simulink model "Final_Report_Carrieri"  (R2020b)
settings: Solver=VariableStepAuto  StartTime=0.0  StopTime=10.0  MaxStep=0.5e-4  RelTol=1e-3
libraries: nesl_utility x12, fl_lib x10, ee_lib x9, simulink x2, powerlib x1
settings Model: Creator=claudio.rossi  LastModifiedBy=lapoc
settings SolverCC: ZeroCrossAlgorithm=Adaptive
settings DebuggingCC: IgnoredZcDiagnostic=none
settings SFSimCC: CustomCodeUndefinedFunction=UseInterfaceOnly

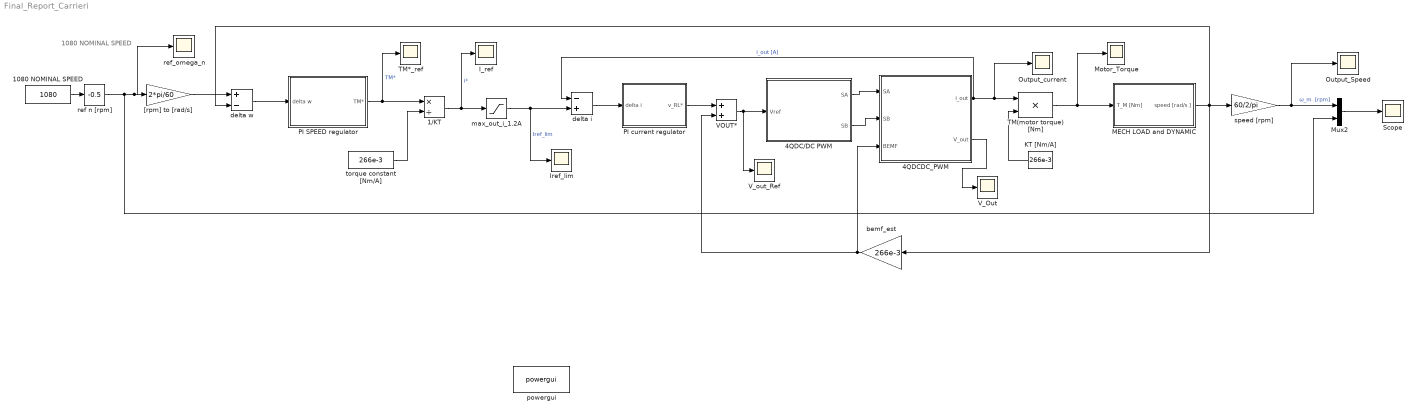
== system Final_Report_Carrieri ==
  note: 1080 NOMINAL SPEED
  1/KT : Product  Inputs=*/
  1080 NOMINAL SPEED : Constant  Value=1080
  4QDC/DC PWM : Subsystem
  4QDCDC_PWM : Subsystem
  I_ref : Scope
  Iref_lim : Scope
  KT [Nm/A] : Constant  Value=266e-3
  MECH LOAD and DYNAMIC : Subsystem
  Motor_Torque : Scope
  Mux2 : Mux  Inputs=2
  Output_Speed : Scope
  Output_current : Scope
  PI SPEED regulator : Subsystem
  PI current regulator : Subsystem
  Scope : Scope
  TM(motor torque) [Nm] : Product
  TM*_ref : Scope
  VOUT* : Sum
  V_Out : Scope
  V_out_Ref : Scope
  "[rpm] to [rad/s]" : Gain  Gain=2*pi/60
  bemf_est : Gain  Gain=266e-3
  delta i : Sum  Inputs=-+
  delta w : Sum  Inputs=+-
  max_out_i_1.2A : Saturate  UpperLimit=1.2  LowerLimit=-1.2
  powergui : powerlib/powergui  Priority=1  SimulationMode=Continuous  SampleTime=50e-6  frequency=60  Iterations=50  frequencyindice=60  Pbase=100e6  ErrMax=1e-4  UnitsV=kV  UnitsW=MW  buscounter=0  FunctionMessages=off  echomessages=off  EnableUseOfTLC=off  CurrentSourceSwitches=off  DisableSnubberDevices=off  DisableRonSwitches=off  DisableVfSwitches=off  DisplayEquations=off  AutomaticDiscreteSolvers=off  SolverType=Tustin/Backward Euler (TBE)  Interpol=off  ExternalGateDelay=off  methode=off  Ts=100  x0status=blocks  SPID=on  SwTol=0  HookPort=off  NonlinearTolerance=1e-4  nMaxIteration=100  ContinueOnMaxIteration=off  RestoreLinks=warning  ResistiveCurrentMeasurement=off  Frange=[0:2:500]  Ylog=off  Xlog=on  ShowGrid=off  save=off  variable=ZData  structure=0  ZoomFFT=off  StartTime=0.0  cycles=1  DisplayStyle=1  fundamental=60  FreqAxis=off  MaxFrequency=1000  frequencyindicesteady=1  RmsSteady=1  display=off
  ref n [rpm] : simulink/Math Operations/Slider Gain  gain=-0.5  low=-1  high=1
  ref_omega_n : Scope
  speed [rpm] : Gain  Gain=60/2/pi
  torque constant [Nm/A] : Constant  Value=266e-3
  wires:
  TM(motor torque) [Nm]/1 -> Motor_Torque/1, MECH LOAD and DYNAMIC/1(T_M [Nm])
  max_out_i_1.2A/1 -> Iref_lim/1, delta i/2  "Iref_lim"
  VOUT*/1 -> V_out_Ref/1, 4QDC/DC PWM/1(Vref)
  ref n [rpm]/1 -> "[rpm] to [rad/s]"/1, ref_omega_n/1, Mux2/2
  Mux2/1 -> Scope/1
  4QDC/DC PWM/2(SB) -> 4QDCDC_PWM/2(SB)
  4QDC/DC PWM/1(SA) -> 4QDCDC_PWM/1(SA)
  KT [Nm/A]/1 -> TM(motor torque) [Nm]/2
  1080 NOMINAL SPEED/1 -> ref n [rpm]/1
  4QDCDC_PWM/2(V_out) -> V_Out/1
  4QDCDC_PWM/1(i_out) -> delta i/1, Output_current/1, TM(motor torque) [Nm]/1  "i_out [A]"
  speed [rpm]/1 -> Output_Speed/1, Mux2/1  "ω_m  [rpm]"
  1/KT/1 -> max_out_i_1.2A/1, I_ref/1  "i*"
  torque constant [Nm/A]/1 -> 1/KT/2
  "[rpm] to [rad/s]"/1 -> delta w/1
  PI SPEED regulator/1(TM*) -> TM*_ref/1, 1/KT/1  "TM*"
  MECH LOAD and DYNAMIC/1(speed [rad/s ]) -> bemf_est/1, speed [rpm]/1, delta w/2
  delta w/1 -> PI SPEED regulator/1(delta w)
  bemf_est/1 -> VOUT*/2, 4QDCDC_PWM/3(BEMF)
  delta i/1 -> PI current regulator/1(delta i)
  PI current regulator/1(v_RL*) -> VOUT*/1

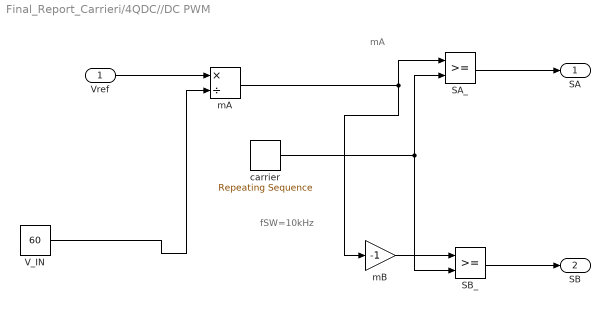
== system Final_Report_Carrieri/4QDC//DC PWM ==
  note: fSW=10kHz
  note: mA
  Vref : Inport
  SA_ : RelationalOperator  OutDataTypeStr=boolean  RndMeth=Simplest
  SB_ : RelationalOperator  OutDataTypeStr=boolean  RndMeth=Simplest
  V_IN : Constant  Value=60
  carrier : simulink/Sources/Repeating Sequence  rep_seq_t=[0 1e-4/2 1e-4]  rep_seq_y=[-1 1 -1]
  mA : Product  Inputs=*/
  mB : Gain  Gain=-1
  SA : Outport  VectorParamsAs1DForOutWhenUnconnected=off
  SB : Outport  Port=2  VectorParamsAs1DForOutWhenUnconnected=off
  wires:
  V_IN/1 -> mA/2
  Vref/1 -> mA/1
  carrier/1 -> SB_/2, SA_/2
  SB_/1 -> SB/1
  mA/1 -> mB/1, SA_/1
  mB/1 -> SB_/1
  SA_/1 -> SA/1

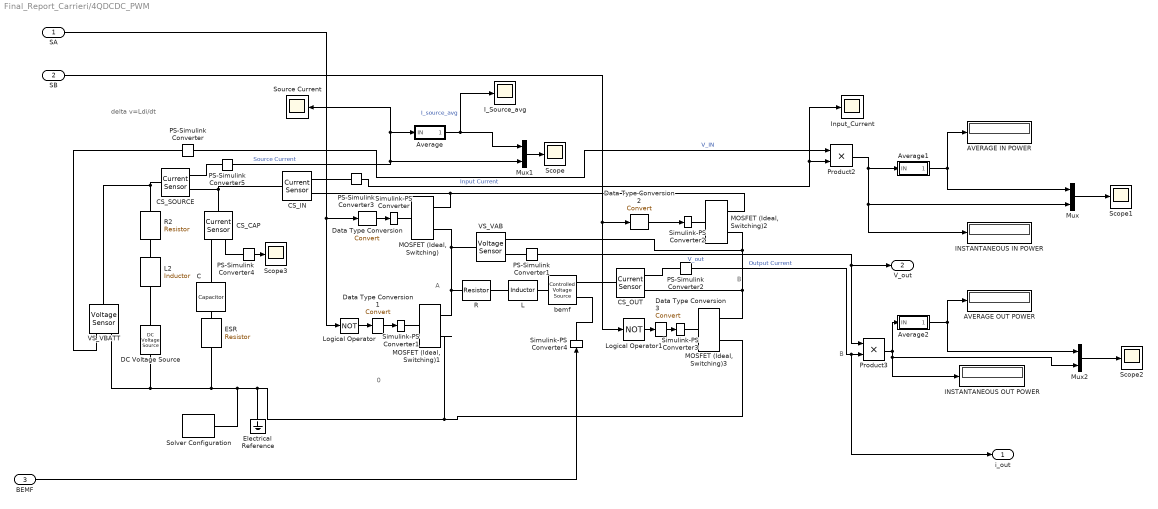
== system Final_Report_Carrieri/4QDCDC_PWM ==
  note: delta v=Ldi/dt
  note: B
  note: 0
  note: A
  note: B
  SA : Inport
  SB : Inport  Port=2
  BEMF : Inport  Port=3
  AVERAGE IN POWER : Display
  AVERAGE OUT POWER : Display
  Average : Subsystem  mask{Ts=1e-4/2}
      mask prompts: Ts "period"
  Average1 : Subsystem  mask{Ts=1e-4/2}
      mask prompts: Ts "period"
  Average2 : Subsystem  mask{Ts=1e-4/2}
      mask prompts: Ts "period"
  C : fl_lib/Electrical/Electrical Elements/Capacitor  c=10 mF  r=1e-9 Ohm  g=0 1/Ohm  i_specify=off  i_priority=None  i=0 A  i_nominal_specify=off  i_nominal_unit=A  i_nominal_value=1  v_specify=off  v_priority=None  v=0 V  v_nominal_specify=off  v_nominal_unit=V  v_nominal_value=1  vc_specify=off  vc_priority=High  vc=0 V  vc_nominal_specify=off  vc_nominal_unit=V  vc_nominal_value=1
  CS_CAP : fl_lib/Electrical/Electrical Sensors/Current Sensor
  CS_IN : fl_lib/Electrical/Electrical Sensors/Current Sensor
  CS_OUT : fl_lib/Electrical/Electrical Sensors/Current Sensor
  CS_SOURCE : fl_lib/Electrical/Electrical Sensors/Current Sensor
  DC Voltage Source : fl_lib/Electrical/Electrical Sources/DC Voltage Source  v0=60 V
  Data Type Conversion{,1..3} (4 alike) : DataTypeConversion
  ESR : ee_lib/Passive/Resistor  R=0.01 Ohm  R_tol=5  enable_R_tol=0  tol_distribution=1  nSigma=4  enable_operating_limits=0  operating_limit_action=2  max_working_voltage=100 V  power_rating=1 W  enable_faults=0  fault_action=1  R_faulted=inf Ohm  enable_temporal_fault=0  t_fault=1 s  enable_behavioral_fault=0  max_permissible_current=1 A  t_fail_on_current=1 s  noise_mode=0  sample_time=1e-3 s  repeatability=1  auto_seed=3499211588  user_seed=0  Tdevice=25 degC  alpha=3.93e-3 1/K  Tmeas=25 degC  thermal_mass=100 J/K  power_derating_T1=70 degC  power_derating_T2=155 degC  operating_temperature_range_vec=[-50, 150] degC  temperature_specify=off  temperature_priority=High  temperature=298.15 K  temperature_nominal_specify=off  temperature_nominal_unit=K  temperature_nominal_value=1
  Electrical Reference : fl_lib/Electrical/Electrical Elements/Electrical Reference
  INSTANTANEOUS IN POWER : Display
  INSTANTANEOUS OUT POWER : Display
  I_Source_avg : Scope
  Input_Current : Scope
  L : ee_lib/Passive/Inductor  l=6.4e-3 H  L_tol=20  enable_L_tol=0  tol_distribution=1  nSigma=4  r=0 Ohm  g=1e-9 1/Ohm  enable_operating_limits=0  operating_limit_action=2  max_working_current=1 A  power_rating=1 W  enable_faults=0  fault_action=1  lambdaPercent=50  k_faulted=0.9999  turnsShort=0  openCct=0  groundShort=0  groundShortG=0 1/Ohm  tau_fault=1e-3 s  enable_temporal_fault=0  t_fault=1 s  enable_behavioral_fault=0  max_permissible_voltage=100 V  n_fail_on_voltage=1  max_permissible_current=1 A  t_fail_on_current=1 s  i_L_specify=off  i_L_priority=High  i_L=0 A  i_L_nominal_specify=off  i_L_nominal_unit=A  i_L_nominal_value=1
  L2 : ee_lib/Passive/Inductor  l=0.6 mH  L_tol=5  enable_L_tol=0  tol_distribution=1  nSigma=4  r=0 Ohm  g=1e-6 1/Ohm  enable_operating_limits=0  operating_limit_action=2  max_working_current=1 A  power_rating=1 W  enable_faults=0  fault_action=1  lambdaPercent=50  k_faulted=0.9999  turnsShort=0  openCct=0  groundShort=0  groundShortG=0 1/Ohm  tau_fault=1e-3 s  enable_temporal_fault=0  t_fault=1 s  enable_behavioral_fault=0  max_permissible_voltage=100 V  n_fail_on_voltage=1  max_permissible_current=1 A  t_fail_on_current=1 s  i_L_specify=off  i_L_priority=High  i_L=0 A  i_L_nominal_specify=off  i_L_nominal_unit=A  i_L_nominal_value=1
  Logical Operator : Logic  Operator=NOT  AllPortsSameDT=off  OutDataTypeStr=boolean
  Logical Operator1 : Logic  Operator=NOT  AllPortsSameDT=off  OutDataTypeStr=boolean
  MOSFET (Ideal, Switching){,1..3} (4 alike) : ee_lib/Semiconductors & Converters/MOSFET (Ideal, Switching)  Rds=0.1 Ohm  Goff=1e-6 1/Ohm  Vth=0.5 V  diode_param=1  diode_Vf=0.8 V  diode_Ron=0.001 Ohm  diode_Goff=1e-5 1/Ohm  diode_C=50e-9 F  diode_iRM=-235 A  diode_iF=300 A  diode_idot=-50 A/us  diode_trr_param=1  diode_trr_factor=3  diode_trr=15 us  diode_Qrr=1500 s*uA  thermal_loss_option=2  Von_data=[0, 1.1, 1.3, 1.45, 1.75, 2.25, 2.7; 0, 1, 1.15, 1.35, 1.7, 2.35, 3] V  Eon_data=[0, .29, 1.43, 2.86, 5.71, 13.14, 22.86; 0, .57, 2.63, 5.14, 10.29, 20.57, 30.29] * 1e-3 J  Eoff_data=[0, .21, 1.07, 2.14, 4.29, 9.86, 17.14; 0, .43, 1.97, 3.86, 7.71, 15.43, 22.71] * 1e-3 J  Tj=[298.15, 398.15] K  Iout_data=[0, 10, 50, 100, 200, 400, 600] A  Eon_scalar=22.86e-3 J  Eoff_scalar=17.14e-3 J  Voff=300 V  Iout_scalar=600 A  diodeModelType=ee.enum.converters.diodeModelType.pwl  diode_IfMat=[.07, .12, .19, 1.75, 4.24, 7.32, 11.2; .16, .3, .72, 2.14, 4.02, 6.35, 9.12] A  diode_TjVec=[25, 125] degC  diode_VfVec=[.5, .7, .9, 1.3, 1.7, 2.1, 2.5] V  thermal_network_parameterization=ee.enum.thermalNetworkTopology.external  Rth=[.03, .2] K/W  Rth_Foster=[.03, .2] K/W  thermal_mass_parameterization=ee.enum.thermalNetwork.timeconstant  thermal_mass=[3, 25] J/K  thermal_mass_Foster=[33, 50] J/K  thermal_time_constant=[.1, 5] s  thermal_time_constant_Foster=[1, 10] s  thermal_mass_initial_temperatures=[25, 25] degC  junction_thermal_mass=0.1 J/K  Tau=1e-4 s  vT_specify=off  vT_priority=None  vT=0 V  vT_nominal_specify=off  vT_nominal_unit=V  vT_nominal_value=1  Qj_specify=off  Qj_priority=None  Qj=0 W  Qj_nominal_specify=off  Qj_nominal_unit=W  Qj_nominal_value=1  junction_temperature_specify=off  junction_temperature_priority=None  junction_temperature=25 degC  junction_temperature_nominal_specify=off  junction_temperature_nominal_unit=degC  junction_temperature_nominal_value=1
  Mux : Mux  Inputs=2
  Mux1 : Mux  Inputs=2
  Mux2 : Mux  Inputs=2
  PS-Simulink Converter{,1..5} (6 alike) : nesl_utility/PS-Simulink Converter  PhysicalDomain=network_engine_domain  SubClassName=ps_output  LeftPortType=input  RightPortType=output  PseudoPeriodic=off  Frequencies=[]  Unit=1  AffineConversion=off
  Product2 : Product
  Product3 : Product
  R : ee_lib/Passive/Resistor  R=24.9 Ohm  R_tol=5  enable_R_tol=0  tol_distribution=1  nSigma=4  enable_operating_limits=0  operating_limit_action=2  max_working_voltage=100 V  power_rating=1 W  enable_faults=0  fault_action=1  R_faulted=inf Ohm  enable_temporal_fault=0  t_fault=1 s  enable_behavioral_fault=0  max_permissible_current=1 A  t_fail_on_current=1 s  noise_mode=0  sample_time=1e-3 s  repeatability=1  auto_seed=3890346746  user_seed=0  Tdevice=25 degC  alpha=3.93e-3 1/K  Tmeas=25 degC  thermal_mass=100 J/K  power_derating_T1=70 degC  power_derating_T2=155 degC  operating_temperature_range_vec=[-50, 150] degC  temperature_specify=off  temperature_priority=High  temperature=298.15 K  temperature_nominal_specify=off  temperature_nominal_unit=K  temperature_nominal_value=1
  R2 : ee_lib/Passive/Resistor  R=0.60 Ohm  R_tol=1  enable_R_tol=0  tol_distribution=1  nSigma=4  enable_operating_limits=0  operating_limit_action=2  max_working_voltage=100 V  power_rating=1 W  enable_faults=0  fault_action=1  R_faulted=inf Ohm  enable_temporal_fault=0  t_fault=1 s  enable_behavioral_fault=0  max_permissible_current=1 A  t_fail_on_current=1 s  noise_mode=0  sample_time=1e-3 s  repeatability=1  auto_seed=545404223  user_seed=0  Tdevice=25 degC  alpha=3.93e-3 1/K  Tmeas=25 degC  thermal_mass=100 J/K  power_derating_T1=70 degC  power_derating_T2=155 degC  operating_temperature_range_vec=[-50, 150] degC  temperature_specify=off  temperature_priority=High  temperature=298.15 K  temperature_nominal_specify=off  temperature_nominal_unit=K  temperature_nominal_value=1
  Scope{,1..3} (4 alike) : Scope
  Simulink-PS Converter{,1..4} (5 alike) : nesl_utility/Simulink-PS Converter  PhysicalDomain=network_engine_domain  SubClassName=ps_input  LeftPortType=input  RightPortType=output  PseudoPeriodic=off  Frequencies=[]  NoiseDistribution=none  NoiseParameters=[]  Unit=1  AffineConversion=off  FilteringAndDerivatives=provide  SimscapeFilterOrder=1  InputFilterTimeConstant=0.001  UdotUserProvided=0
  Solver Configuration : nesl_utility/Solver Configuration  PhysicalDomain=network_engine_domain  SubClassName=solver  LeftPortType=input  RightPortType=generic  Tones=[]  Harmonics=[]  SimulateNoise=off  Profile=off  UseLocalSampling=off  EnableSwitchedLinearOptims=on  FrequencyDomain=off  UseCCode=off  RelTol=0.001  AbsTol=1e-06  MinStep=1e-09  ToWorkspace=off  RevertToSquareIcSolve=off  NumHomotopyIterations=100  PhasorMode=off  PhasorModeNumHarmonics=1  DoDC=off  ResidualTolerance=1e-09  UseLocalSolver=off  LocalSolverChoice=NE_BACKWARD_EULER_ADVANCER  LocalSolverSampleTime=0.001  DoFixedCost=off  MaxNonlinIter=3  MaxModeIter=2  ComputeImpulses=off  ImpulseIterations=2  LinearAlgebra=auto  EquationFormulation=NE_TIME_EF  DelaysMemoryBudget=1024  AutomaticFiltering=on  FilteringTimeConstant=0.001  PartitionStorageMethod=AS_NEEDED  PartitionMemoryBudget=1024  PartitionMethod=ROBUST
  Source Current : Scope
  VS_VAB : fl_lib/Electrical/Electrical Sensors/Voltage Sensor
  VS_VBATT : fl_lib/Electrical/Electrical Sensors/Voltage Sensor
  bemf : fl_lib/Electrical/Electrical Sources/Controlled Voltage Source
  i_out : Outport  VectorParamsAs1DForOutWhenUnconnected=off
  V_out : Outport  Port=2  VectorParamsAs1DForOutWhenUnconnected=off
  wires:
  BEMF/1 -> Simulink-PS Converter4/1
  Data Type Conversion3/1 -> Simulink-PS Converter3/1
  Logical Operator/1 -> Data Type Conversion1/1
  SA/1 -> Logical Operator/1, Data Type Conversion/1
  SB/1 -> Data Type Conversion2/1, Logical Operator1/1
  Data Type Conversion/1 -> Simulink-PS Converter/1
  Data Type Conversion1/1 -> Simulink-PS Converter1/1
  Logical Operator1/1 -> Data Type Conversion3/1
  Data Type Conversion2/1 -> Simulink-PS Converter2/1
  Product2/1 -> Mux/2, INSTANTANEOUS IN POWER/1, Average1/1(IN)
  PS-Simulink Converter1/1 -> Product3/1, V_out/1  "V_out"
  Average1/1(OUT) -> AVERAGE IN POWER/1, Mux/1
  PS-Simulink Converter2/1 -> i_out/1, Product3/2  "Output Current"
  Product3/1 -> Average2/1(IN), INSTANTANEOUS OUT POWER/1, Mux2/2
  Average2/1(OUT) -> Mux2/1, AVERAGE OUT POWER/1
  Mux1/1 -> Scope/1
  Average/1(OUT) -> I_Source_avg/1, Mux1/1  "I_source_avg"
  PS-Simulink Converter5/1 -> Source Current/1, Average/1(IN), Mux1/2  "Source Current"
  PS-Simulink Converter/1 -> Product2/1  "V_IN"
  PS-Simulink Converter3/1 -> Input_Current/1, Product2/2  "Input Current"
  Mux2/1 -> Scope2/1
  Mux/1 -> Scope1/1
  PS-Simulink Converter4/1 -> Scope3/1
  connections:
  Simulink-PS Converter1/RConn1 -- "MOSFET (Ideal, Switching)1"/LConn1
  "MOSFET (Ideal, Switching)3"/RConn2 -- "MOSFET (Ideal, Switching)1"/RConn2 -- Electrical Reference/LConn1 -- VS_VBATT/RConn2 -- DC Voltage Source/RConn1 -- ESR/RConn1 -- Solver Configuration/RConn1
  CS_IN/LConn1 -- CS_SOURCE/RConn2 -- CS_CAP/LConn1
  CS_IN/RConn1 -- PS-Simulink Converter3/LConn1
  "MOSFET (Ideal, Switching)"/RConn2 -- R/LConn1 -- "MOSFET (Ideal, Switching)1"/RConn1 -- VS_VAB/LConn1
  CS_OUT/RConn1 -- PS-Simulink Converter2/LConn1
  bemf/LConn1 -- L/RConn1
  VS_VBATT/RConn1 -- PS-Simulink Converter/LConn1
  Simulink-PS Converter2/RConn1 -- "MOSFET (Ideal, Switching)2"/LConn1
  "MOSFET (Ideal, Switching)2"/RConn2 -- VS_VAB/RConn2 -- "MOSFET (Ideal, Switching)3"/RConn1 -- CS_OUT/RConn2
  bemf/RConn2 -- CS_OUT/LConn1
  CS_IN/RConn2 -- "MOSFET (Ideal, Switching)2"/RConn1 -- "MOSFET (Ideal, Switching)"/RConn1
  L/LConn1 -- R/RConn1
  Simulink-PS Converter4/RConn1 -- bemf/RConn1
  Simulink-PS Converter/RConn1 -- "MOSFET (Ideal, Switching)"/LConn1
  PS-Simulink Converter1/LConn1 -- VS_VAB/RConn1
  Simulink-PS Converter3/RConn1 -- "MOSFET (Ideal, Switching)3"/LConn1
  DC Voltage Source/LConn1 -- L2/RConn1
  L2/LConn1 -- R2/RConn1
  C/RConn1 -- ESR/LConn1
  C/LConn1 -- CS_CAP/RConn2
  R2/LConn1 -- CS_SOURCE/LConn1 -- VS_VBATT/LConn1
  CS_CAP/RConn1 -- PS-Simulink Converter4/LConn1
  PS-Simulink Converter5/LConn1 -- CS_SOURCE/RConn1

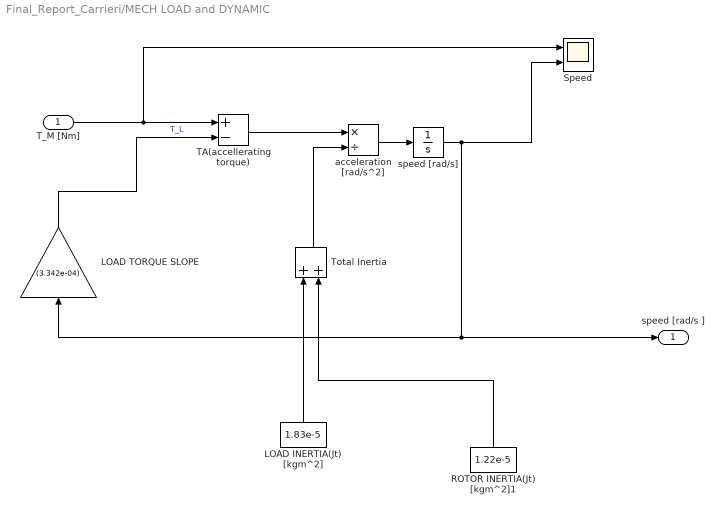
== system Final_Report_Carrieri/MECH LOAD and DYNAMIC ==
  T_M [Nm] : Inport
  LOAD INERTIA(Jt) [kgm^2] : Constant  Value=1.83e-5
  LOAD TORQUE SLOPE : Gain  Gain=(3.342e-04)
  ROTOR INERTIA(Jt) [kgm^2]1 : Constant  Value=1.22e-5
  Speed : Scope  NumInputPorts=2
  TA(accellerating torque) : Sum  Inputs=+-
  Total Inertia : Sum
  acceleration [rad/s^2] : Product  Inputs=*/
  speed [rad/s] : Integrator
  speed [rad/s ] : Outport  VectorParamsAs1DForOutWhenUnconnected=off
  wires:
  LOAD INERTIA(Jt) [kgm^2]/1 -> Total Inertia/1
  speed [rad/s]/1 -> LOAD TORQUE SLOPE/1, speed [rad/s ]/1, Speed/2
  TA(accellerating torque)/1 -> acceleration [rad/s^2]/1
  acceleration [rad/s^2]/1 -> speed [rad/s]/1
  T_M [Nm]/1 -> Speed/1, TA(accellerating torque)/1
  LOAD TORQUE SLOPE/1 -> TA(accellerating torque)/2  "T_L"
  Total Inertia/1 -> acceleration [rad/s^2]/2
  ROTOR INERTIA(Jt) [kgm^2]1/1 -> Total Inertia/2

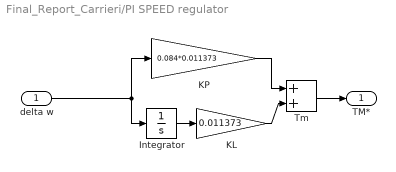
== system Final_Report_Carrieri/PI SPEED regulator ==
  delta w : Inport
  Integrator : Integrator
  KL : Gain  Gain=0.011373
  KP : Gain  Gain=0.084*0.011373
  Tm : Sum
  TM* : Outport  VectorParamsAs1DForOutWhenUnconnected=off
  wires:
  Tm/1 -> TM*/1
  Integrator/1 -> KL/1
  KL/1 -> Tm/2
  delta w/1 -> KP/1, Integrator/1
  KP/1 -> Tm/1

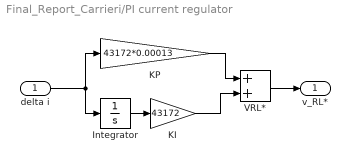
== system Final_Report_Carrieri/PI current regulator ==
  delta i : Inport
  Integrator : Integrator
  KI : Gain  Gain=43172
  KP : Gain  Gain=43172*0.00013
  VRL* : Sum
  v_RL* : Outport  VectorParamsAs1DForOutWhenUnconnected=off
  wires:
  KP/1 -> VRL*/1
  delta i/1 -> Integrator/1, KP/1
  KI/1 -> VRL*/2
  Integrator/1 -> KI/1
  VRL*/1 -> v_RL*/1

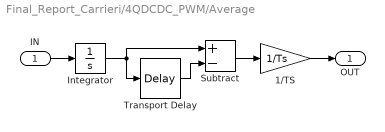
== system Final_Report_Carrieri/4QDCDC_PWM/Average ==
  IN : Inport
  1/TS : Gain  Gain=1/Ts
  Integrator : Integrator
  Subtract : Sum  Inputs=+-
  Transport Delay : TransportDelay  DelayTime=Ts  BufferSize=5120
  OUT : Outport  VectorParamsAs1DForOutWhenUnconnected=off
  wires:
  Integrator/1 -> Transport Delay/1, Subtract/1
  1/TS/1 -> OUT/1
  IN/1 -> Integrator/1
  Transport Delay/1 -> Subtract/2
  Subtract/1 -> 1/TS/1

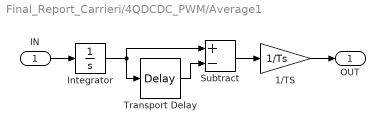
== system Final_Report_Carrieri/4QDCDC_PWM/Average1 ==
  IN : Inport
  1/TS : Gain  Gain=1/Ts
  Integrator : Integrator
  Subtract : Sum  Inputs=+-
  Transport Delay : TransportDelay  DelayTime=Ts  BufferSize=5120
  OUT : Outport  VectorParamsAs1DForOutWhenUnconnected=off
  wires:
  Integrator/1 -> Transport Delay/1, Subtract/1
  1/TS/1 -> OUT/1
  IN/1 -> Integrator/1
  Transport Delay/1 -> Subtract/2
  Subtract/1 -> 1/TS/1

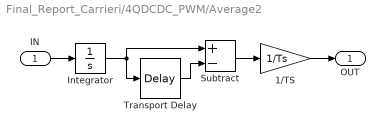
== system Final_Report_Carrieri/4QDCDC_PWM/Average2 ==
  IN : Inport
  1/TS : Gain  Gain=1/Ts
  Integrator : Integrator
  Subtract : Sum  Inputs=+-
  Transport Delay : TransportDelay  DelayTime=Ts  BufferSize=5120
  OUT : Outport  VectorParamsAs1DForOutWhenUnconnected=off
  wires:
  Integrator/1 -> Transport Delay/1, Subtract/1
  1/TS/1 -> OUT/1
  IN/1 -> Integrator/1
  Transport Delay/1 -> Subtract/2
  Subtract/1 -> 1/TS/1
